simulink model "diagonalize"  (R2021a)
settings: Solver=VariableStepAuto  StartTime=0.0  StopTime=10.0  RelTol=1e-3
settings Model: Creator=davidrico  LastModifiedBy=davidrico

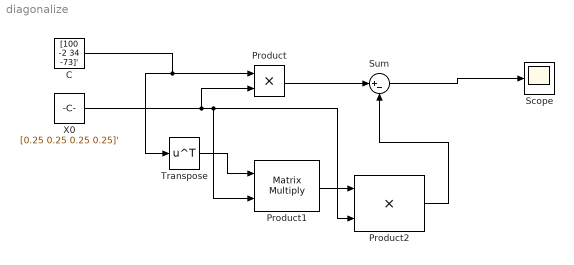
== system diagonalize ==
  C : Constant  Value=[100 -2 34 -73]'
  Product : Product
  Product1 : Product  Multiplication=Matrix(*)
  Product2 : Product
  Scope : Scope
  Sum : Sum  Inputs=|+-
  Transpose : Math  Operator=transpose  SaturateOnIntegerOverflow=on
  X0 : Constant  Value=[0.25 0.25 0.25 0.25]'
  wires:
  C/1 -> Product/1, Transpose/1
  X0/1 -> Product1/2, Product2/2, Product/2
  Product/1 -> Sum/1
  Transpose/1 -> Product1/1
  Product1/1 -> Product2/1
  Product2/1 -> Sum/2
  Sum/1 -> Scope/1
